simulink model "MdXX_RspOutComm1"  (R2018b)
settings: Solver=FixedStepDiscrete  StartTime=0.0  StopTime=10.0  FixedStep=0.01  RelTol=1e-3
undefined symbols (not defined in the file or in its folder): KeSMSuRspStatHldTm_Val, MdRspLocal2, SrcReqTp1
libraries: simulink x64, RspLib x32
(part 1 of 4)
settings Model: Creator=sn2xws  LastModifiedBy=sn2xws
settings Model: ModifiedHistory=|
  | MD2,MD3不反馈问题修复
  | V2.4.0 Bug 692977 7座 行李箱模式，在调用过程中切换挡位打断调用，返回信号有误
  | 2024.8.19 V3.0.0 Md29反馈逻辑更新
  | //2024.8.20 V3.0.1增加Md53,Md56的反馈
  | 2024.9.13 V3.0.1增加Md2，Md3，Md29被中断的反馈BUG 920831,920834
  | 2024.12.18 V3.8.0 CR 955881 <REQ_MSM_868>
settings DataIOCC: SaveFormat=StructureWithTime
settings OptimizationCC: DefaultParameterBehavior=Inlined  EnhancedBackFolding=on  PassReuseOutputArgsAs=Individual arguments  ZeroExternalMemoryAtStartup=off  ZeroInternalMemoryAtStartup=off  OptimizeBlockOrder=speed  DifferentSizesBufferReuse=on  OptimizationCustomize=off
settings DebuggingCC: ParameterTunabilityLossMsg=error
settings ModelReferenceCC: ModelReferenceNumInstancesAllowed=Single
settings SFSimCC: MATLABDynamicMemAlloc=off
settings RTWCC: SystemTargetFile=autosar.tlc  GenCodeOnly=on  TemplateMakefile=ert_default_tmf  Description=AUTOSAR  GenerateReport=on  IncludeHyperlinkInReport=on  LaunchReport=on  GenerateTraceInfo=on  GenerateTraceReport=on  GenerateTraceReportSl=on  GenerateTraceReportSf=on  GenerateTraceReportEml=on  GenerateCodeMetricsReport=on
settings CodeAppCC: ForceParamTrailComments=on  IgnoreCustomStorageClasses=off  OperatorAnnotations=on  SimulinkDataObjDesc=on  SFDataObjDesc=on  InsertBlockDesc=on
settings STFCustomTargetCC: TargetLangStandard=C99 (ISO)  MultiwordLength=256  ParMdlRefBuildCompliant=on  CompOptLevelCompliant=on  IncludeMdlTerminateFcn=off  CombineOutputUpdateFcns=on  SuppressErrorStatus=on  ERTCustomFileBanners=on  SupportNonFinite=off  SupportComplex=off  SupportContinuousTime=off  SupportNonInlinedSFcns=off  RemoveResetFunc=on  MATLABClassNameForMDSCustomization=Simulink.SoftwareTarget.ERTCustomization  AutosarCompliant=on  UseToolchainInfoCompliant=on  LookupTableObjectStructAxisOrder=2,1,3,4,...  LUTObjectStructOrderEvenSpacing=Size,Table,Breakpoints  SystemTargetFile=autosar.tlc
settings ERTTargetCC: TargetLangStandard=C99 (ISO)  ConcurrentExecutionCompliant=off  IncludeMdlTerminateFcn=off  SuppressErrorStatus=on  SupportNonFinite=off  SupportComplex=off  ModelStepFunctionPrototypeControlCompliant=off  CPPClassGenCompliant=off  AutosarCompliant=on  LookupTableObjectStructAxisOrder=2,1,3,4,...  LUTObjectStructOrderEvenSpacing=Size,Table,Breakpoints  InlinedParameterPlacement=NonHierarchical  ERTCustomFileTemplate=example_file_process.tlc  ERTFilePackagingFormat=Compact

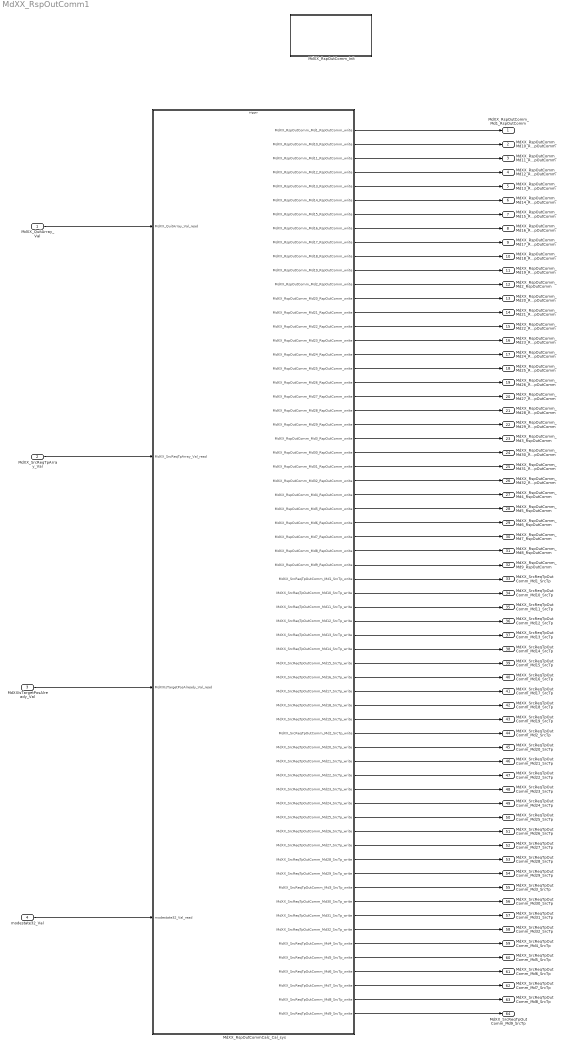
== system MdXX_RspOutComm1 ==
  MdXX_QuitArray_Val : Inport  OutDataTypeStr=Enum: MdRspLocal2  PortDimensions=32
  MdXX_SrcReqTpArray_Val : Inport  Port=2  OutDataTypeStr=Enum: SrcReqTp1  PortDimensions=32
  MdXXIsTargetPosAlready_Val : Inport  Port=3  OutDataTypeStr=uint32  PortDimensions=1
  modestate32_Val : Inport  Port=4  OutDataTypeStr=uint32  PortDimensions=1
  MdXX_RspOutCommCalc_Cal_sys : Subsystem
  MdXX_RspOutComm_Init : Subsystem
  MdXX_RspOutComm_Md1_RspOutComm : Outport  OutDataTypeStr=uint8  PortDimensions=1
  MdXX_RspOutComm_Md10_RspOutComm : Outport  Port=2  OutDataTypeStr=uint8  PortDimensions=1
  MdXX_RspOutComm_Md11_RspOutComm : Outport  Port=3  OutDataTypeStr=uint8  PortDimensions=1
  MdXX_RspOutComm_Md12_RspOutComm : Outport  Port=4  OutDataTypeStr=uint8  PortDimensions=1
  MdXX_RspOutComm_Md13_RspOutComm : Outport  Port=5  OutDataTypeStr=uint8  PortDimensions=1
  MdXX_RspOutComm_Md14_RspOutComm : Outport  Port=6  OutDataTypeStr=uint8  PortDimensions=1
  MdXX_RspOutComm_Md15_RspOutComm : Outport  Port=7  OutDataTypeStr=uint8  PortDimensions=1
  MdXX_RspOutComm_Md16_RspOutComm : Outport  Port=8  OutDataTypeStr=uint8  PortDimensions=1
  MdXX_RspOutComm_Md17_RspOutComm : Outport  Port=9  OutDataTypeStr=uint8  PortDimensions=1
  MdXX_RspOutComm_Md18_RspOutComm : Outport  Port=10  OutDataTypeStr=uint8  PortDimensions=1
  MdXX_RspOutComm_Md19_RspOutComm : Outport  Port=11  OutDataTypeStr=uint8  PortDimensions=1
  MdXX_RspOutComm_Md2_RspOutComm : Outport  Port=12  OutDataTypeStr=uint8  PortDimensions=1
  MdXX_RspOutComm_Md20_RspOutComm : Outport  Port=13  OutDataTypeStr=uint8  PortDimensions=1
  MdXX_RspOutComm_Md21_RspOutComm : Outport  Port=14  OutDataTypeStr=uint8  PortDimensions=1
  MdXX_RspOutComm_Md22_RspOutComm : Outport  Port=15  OutDataTypeStr=uint8  PortDimensions=1
  MdXX_RspOutComm_Md23_RspOutComm : Outport  Port=16  OutDataTypeStr=uint8  PortDimensions=1
  MdXX_RspOutComm_Md24_RspOutComm : Outport  Port=17  OutDataTypeStr=uint8  PortDimensions=1
  MdXX_RspOutComm_Md25_RspOutComm : Outport  Port=18  OutDataTypeStr=uint8  PortDimensions=1
  MdXX_RspOutComm_Md26_RspOutComm : Outport  Port=19  OutDataTypeStr=uint8  PortDimensions=1
  MdXX_RspOutComm_Md27_RspOutComm : Outport  Port=20  OutDataTypeStr=uint8  PortDimensions=1
  MdXX_RspOutComm_Md28_RspOutComm : Outport  Port=21  OutDataTypeStr=uint8  PortDimensions=1
  MdXX_RspOutComm_Md29_RspOutComm : Outport  Port=22  OutDataTypeStr=uint8  PortDimensions=1
  MdXX_RspOutComm_Md3_RspOutComm : Outport  Port=23  OutDataTypeStr=uint8  PortDimensions=1
  MdXX_RspOutComm_Md30_RspOutComm : Outport  Port=24  OutDataTypeStr=uint8  PortDimensions=1
  MdXX_RspOutComm_Md31_RspOutComm : Outport  Port=25  OutDataTypeStr=uint8  PortDimensions=1
  MdXX_RspOutComm_Md32_RspOutComm : Outport  Port=26  OutDataTypeStr=uint8  PortDimensions=1
  MdXX_RspOutComm_Md4_RspOutComm : Outport  Port=27  OutDataTypeStr=uint8  PortDimensions=1
  MdXX_RspOutComm_Md5_RspOutComm : Outport  Port=28  OutDataTypeStr=uint8  PortDimensions=1
  MdXX_RspOutComm_Md6_RspOutComm : Outport  Port=29  OutDataTypeStr=uint8  PortDimensions=1
  MdXX_RspOutComm_Md7_RspOutComm : Outport  Port=30  OutDataTypeStr=uint8  PortDimensions=1
  MdXX_RspOutComm_Md8_RspOutComm : Outport  Port=31  OutDataTypeStr=uint8  PortDimensions=1
  MdXX_RspOutComm_Md9_RspOutComm : Outport  Port=32  OutDataTypeStr=uint8  PortDimensions=1
  MdXX_SrcReqTpOutComm_Md1_SrcTp : Outport  Port=33  OutDataTypeStr=Enum: SrcReqTp1  PortDimensions=1
  MdXX_SrcReqTpOutComm_Md10_SrcTp : Outport  Port=34  OutDataTypeStr=Enum: SrcReqTp1  PortDimensions=1
  MdXX_SrcReqTpOutComm_Md11_SrcTp : Outport  Port=35  OutDataTypeStr=Enum: SrcReqTp1  PortDimensions=1
  MdXX_SrcReqTpOutComm_Md12_SrcTp : Outport  Port=36  OutDataTypeStr=Enum: SrcReqTp1  PortDimensions=1
  MdXX_SrcReqTpOutComm_Md13_SrcTp : Outport  Port=37  OutDataTypeStr=Enum: SrcReqTp1  PortDimensions=1
  MdXX_SrcReqTpOutComm_Md14_SrcTp : Outport  Port=38  OutDataTypeStr=Enum: SrcReqTp1  PortDimensions=1
  MdXX_SrcReqTpOutComm_Md15_SrcTp : Outport  Port=39  OutDataTypeStr=Enum: SrcReqTp1  PortDimensions=1
  MdXX_SrcReqTpOutComm_Md16_SrcTp : Outport  Port=40  OutDataTypeStr=Enum: SrcReqTp1  PortDimensions=1
  MdXX_SrcReqTpOutComm_Md17_SrcTp : Outport  Port=41  OutDataTypeStr=Enum: SrcReqTp1  PortDimensions=1
  MdXX_SrcReqTpOutComm_Md18_SrcTp : Outport  Port=42  OutDataTypeStr=Enum: SrcReqTp1  PortDimensions=1
  MdXX_SrcReqTpOutComm_Md19_SrcTp : Outport  Port=43  OutDataTypeStr=Enum: SrcReqTp1  PortDimensions=1
  MdXX_SrcReqTpOutComm_Md2_SrcTp : Outport  Port=44  OutDataTypeStr=Enum: SrcReqTp1  PortDimensions=1
  MdXX_SrcReqTpOutComm_Md20_SrcTp : Outport  Port=45  OutDataTypeStr=Enum: SrcReqTp1  PortDimensions=1
  MdXX_SrcReqTpOutComm_Md21_SrcTp : Outport  Port=46  OutDataTypeStr=Enum: SrcReqTp1  PortDimensions=1
  MdXX_SrcReqTpOutComm_Md22_SrcTp : Outport  Port=47  OutDataTypeStr=Enum: SrcReqTp1  PortDimensions=1
  MdXX_SrcReqTpOutComm_Md23_SrcTp : Outport  Port=48  OutDataTypeStr=Enum: SrcReqTp1  PortDimensions=1
  MdXX_SrcReqTpOutComm_Md24_SrcTp : Outport  Port=49  OutDataTypeStr=Enum: SrcReqTp1  PortDimensions=1
  MdXX_SrcReqTpOutComm_Md25_SrcTp : Outport  Port=50  OutDataTypeStr=Enum: SrcReqTp1  PortDimensions=1
  MdXX_SrcReqTpOutComm_Md26_SrcTp : Outport  Port=51  OutDataTypeStr=Enum: SrcReqTp1  PortDimensions=1
  MdXX_SrcReqTpOutComm_Md27_SrcTp : Outport  Port=52  OutDataTypeStr=Enum: SrcReqTp1  PortDimensions=1
  MdXX_SrcReqTpOutComm_Md28_SrcTp : Outport  Port=53  OutDataTypeStr=Enum: SrcReqTp1  PortDimensions=1
  MdXX_SrcReqTpOutComm_Md29_SrcTp : Outport  Port=54  OutDataTypeStr=Enum: SrcReqTp1  PortDimensions=1
  MdXX_SrcReqTpOutComm_Md3_SrcTp : Outport  Port=55  OutDataTypeStr=Enum: SrcReqTp1  PortDimensions=1
  MdXX_SrcReqTpOutComm_Md30_SrcTp : Outport  Port=56  OutDataTypeStr=Enum: SrcReqTp1  PortDimensions=1
  MdXX_SrcReqTpOutComm_Md31_SrcTp : Outport  Port=57  OutDataTypeStr=Enum: SrcReqTp1  PortDimensions=1
  MdXX_SrcReqTpOutComm_Md32_SrcTp : Outport  Port=58  OutDataTypeStr=Enum: SrcReqTp1  PortDimensions=1
  MdXX_SrcReqTpOutComm_Md4_SrcTp : Outport  Port=59  OutDataTypeStr=Enum: SrcReqTp1  PortDimensions=1
  MdXX_SrcReqTpOutComm_Md5_SrcTp : Outport  Port=60  OutDataTypeStr=Enum: SrcReqTp1  PortDimensions=1
  MdXX_SrcReqTpOutComm_Md6_SrcTp : Outport  Port=61  OutDataTypeStr=Enum: SrcReqTp1  PortDimensions=1
  MdXX_SrcReqTpOutComm_Md7_SrcTp : Outport  Port=62  OutDataTypeStr=Enum: SrcReqTp1  PortDimensions=1
  MdXX_SrcReqTpOutComm_Md8_SrcTp : Outport  Port=63  OutDataTypeStr=Enum: SrcReqTp1  PortDimensions=1
  MdXX_SrcReqTpOutComm_Md9_SrcTp : Outport  Port=64  OutDataTypeStr=Enum: SrcReqTp1  PortDimensions=1
  wires:
  MdXX_QuitArray_Val/1 -> MdXX_RspOutCommCalc_Cal_sys/1(MdXX_QuitArray_Val_read)
  MdXX_SrcReqTpArray_Val/1 -> MdXX_RspOutCommCalc_Cal_sys/2(MdXX_SrcReqTpArray_Val_read)
  modestate32_Val/1 -> MdXX_RspOutCommCalc_Cal_sys/4(modestate32_Val_read)
  MdXXIsTargetPosAlready_Val/1 -> MdXX_RspOutCommCalc_Cal_sys/3(MdXXIsTargetPosAlready_Val_read)
  MdXX_RspOutCommCalc_Cal_sys/1(MdXX_RspOutComm_Md1_RspOutComm_write) -> MdXX_RspOutComm_Md1_RspOutComm/1
  MdXX_RspOutCommCalc_Cal_sys/2(MdXX_RspOutComm_Md10_RspOutComm_write) -> MdXX_RspOutComm_Md10_RspOutComm/1
  MdXX_RspOutCommCalc_Cal_sys/3(MdXX_RspOutComm_Md11_RspOutComm_write) -> MdXX_RspOutComm_Md11_RspOutComm/1
  MdXX_RspOutCommCalc_Cal_sys/4(MdXX_RspOutComm_Md12_RspOutComm_write) -> MdXX_RspOutComm_Md12_RspOutComm/1
  MdXX_RspOutCommCalc_Cal_sys/5(MdXX_RspOutComm_Md13_RspOutComm_write) -> MdXX_RspOutComm_Md13_RspOutComm/1
  MdXX_RspOutCommCalc_Cal_sys/6(MdXX_RspOutComm_Md14_RspOutComm_write) -> MdXX_RspOutComm_Md14_RspOutComm/1
  MdXX_RspOutCommCalc_Cal_sys/7(MdXX_RspOutComm_Md15_RspOutComm_write) -> MdXX_RspOutComm_Md15_RspOutComm/1
  MdXX_RspOutCommCalc_Cal_sys/8(MdXX_RspOutComm_Md16_RspOutComm_write) -> MdXX_RspOutComm_Md16_RspOutComm/1
  MdXX_RspOutCommCalc_Cal_sys/9(MdXX_RspOutComm_Md17_RspOutComm_write) -> MdXX_RspOutComm_Md17_RspOutComm/1
  MdXX_RspOutCommCalc_Cal_sys/10(MdXX_RspOutComm_Md18_RspOutComm_write) -> MdXX_RspOutComm_Md18_RspOutComm/1
  MdXX_RspOutCommCalc_Cal_sys/11(MdXX_RspOutComm_Md19_RspOutComm_write) -> MdXX_RspOutComm_Md19_RspOutComm/1
  MdXX_RspOutCommCalc_Cal_sys/12(MdXX_RspOutComm_Md2_RspOutComm_write) -> MdXX_RspOutComm_Md2_RspOutComm/1
  MdXX_RspOutCommCalc_Cal_sys/13(MdXX_RspOutComm_Md20_RspOutComm_write) -> MdXX_RspOutComm_Md20_RspOutComm/1
  MdXX_RspOutCommCalc_Cal_sys/14(MdXX_RspOutComm_Md21_RspOutComm_write) -> MdXX_RspOutComm_Md21_RspOutComm/1
  MdXX_RspOutCommCalc_Cal_sys/15(MdXX_RspOutComm_Md22_RspOutComm_write) -> MdXX_RspOutComm_Md22_RspOutComm/1
  MdXX_RspOutCommCalc_Cal_sys/16(MdXX_RspOutComm_Md23_RspOutComm_write) -> MdXX_RspOutComm_Md23_RspOutComm/1
  MdXX_RspOutCommCalc_Cal_sys/17(MdXX_RspOutComm_Md24_RspOutComm_write) -> MdXX_RspOutComm_Md24_RspOutComm/1
  MdXX_RspOutCommCalc_Cal_sys/18(MdXX_RspOutComm_Md25_RspOutComm_write) -> MdXX_RspOutComm_Md25_RspOutComm/1
  MdXX_RspOutCommCalc_Cal_sys/19(MdXX_RspOutComm_Md26_RspOutComm_write) -> MdXX_RspOutComm_Md26_RspOutComm/1
  MdXX_RspOutCommCalc_Cal_sys/20(MdXX_RspOutComm_Md27_RspOutComm_write) -> MdXX_RspOutComm_Md27_RspOutComm/1
  MdXX_RspOutCommCalc_Cal_sys/21(MdXX_RspOutComm_Md28_RspOutComm_write) -> MdXX_RspOutComm_Md28_RspOutComm/1
  MdXX_RspOutCommCalc_Cal_sys/22(MdXX_RspOutComm_Md29_RspOutComm_write) -> MdXX_RspOutComm_Md29_RspOutComm/1
  MdXX_RspOutCommCalc_Cal_sys/23(MdXX_RspOutComm_Md3_RspOutComm_write) -> MdXX_RspOutComm_Md3_RspOutComm/1
  MdXX_RspOutCommCalc_Cal_sys/24(MdXX_RspOutComm_Md30_RspOutComm_write) -> MdXX_RspOutComm_Md30_RspOutComm/1
  MdXX_RspOutCommCalc_Cal_sys/25(MdXX_RspOutComm_Md31_RspOutComm_write) -> MdXX_RspOutComm_Md31_RspOutComm/1
  MdXX_RspOutCommCalc_Cal_sys/26(MdXX_RspOutComm_Md32_RspOutComm_write) -> MdXX_RspOutComm_Md32_RspOutComm/1
  MdXX_RspOutCommCalc_Cal_sys/27(MdXX_RspOutComm_Md4_RspOutComm_write) -> MdXX_RspOutComm_Md4_RspOutComm/1
  MdXX_RspOutCommCalc_Cal_sys/28(MdXX_RspOutComm_Md5_RspOutComm_write) -> MdXX_RspOutComm_Md5_RspOutComm/1
  MdXX_RspOutCommCalc_Cal_sys/29(MdXX_RspOutComm_Md6_RspOutComm_write) -> MdXX_RspOutComm_Md6_RspOutComm/1
  MdXX_RspOutCommCalc_Cal_sys/30(MdXX_RspOutComm_Md7_RspOutComm_write) -> MdXX_RspOutComm_Md7_RspOutComm/1
  MdXX_RspOutCommCalc_Cal_sys/31(MdXX_RspOutComm_Md8_RspOutComm_write) -> MdXX_RspOutComm_Md8_RspOutComm/1
  MdXX_RspOutCommCalc_Cal_sys/32(MdXX_RspOutComm_Md9_RspOutComm_write) -> MdXX_RspOutComm_Md9_RspOutComm/1
  MdXX_RspOutCommCalc_Cal_sys/33(MdXX_SrcReqTpOutComm_Md1_SrcTp_write) -> MdXX_SrcReqTpOutComm_Md1_SrcTp/1
  MdXX_RspOutCommCalc_Cal_sys/34(MdXX_SrcReqTpOutComm_Md10_SrcTp_write) -> MdXX_SrcReqTpOutComm_Md10_SrcTp/1
  MdXX_RspOutCommCalc_Cal_sys/35(MdXX_SrcReqTpOutComm_Md11_SrcTp_write) -> MdXX_SrcReqTpOutComm_Md11_SrcTp/1
  MdXX_RspOutCommCalc_Cal_sys/36(MdXX_SrcReqTpOutComm_Md12_SrcTp_write) -> MdXX_SrcReqTpOutComm_Md12_SrcTp/1
  MdXX_RspOutCommCalc_Cal_sys/37(MdXX_SrcReqTpOutComm_Md13_SrcTp_write) -> MdXX_SrcReqTpOutComm_Md13_SrcTp/1
  MdXX_RspOutCommCalc_Cal_sys/38(MdXX_SrcReqTpOutComm_Md14_SrcTp_write) -> MdXX_SrcReqTpOutComm_Md14_SrcTp/1
  MdXX_RspOutCommCalc_Cal_sys/39(MdXX_SrcReqTpOutComm_Md15_SrcTp_write) -> MdXX_SrcReqTpOutComm_Md15_SrcTp/1
  MdXX_RspOutCommCalc_Cal_sys/40(MdXX_SrcReqTpOutComm_Md16_SrcTp_write) -> MdXX_SrcReqTpOutComm_Md16_SrcTp/1
  MdXX_RspOutCommCalc_Cal_sys/41(MdXX_SrcReqTpOutComm_Md17_SrcTp_write) -> MdXX_SrcReqTpOutComm_Md17_SrcTp/1
  MdXX_RspOutCommCalc_Cal_sys/42(MdXX_SrcReqTpOutComm_Md18_SrcTp_write) -> MdXX_SrcReqTpOutComm_Md18_SrcTp/1
  MdXX_RspOutCommCalc_Cal_sys/43(MdXX_SrcReqTpOutComm_Md19_SrcTp_write) -> MdXX_SrcReqTpOutComm_Md19_SrcTp/1
  MdXX_RspOutCommCalc_Cal_sys/44(MdXX_SrcReqTpOutComm_Md2_SrcTp_write) -> MdXX_SrcReqTpOutComm_Md2_SrcTp/1
  MdXX_RspOutCommCalc_Cal_sys/45(MdXX_SrcReqTpOutComm_Md20_SrcTp_write) -> MdXX_SrcReqTpOutComm_Md20_SrcTp/1
  MdXX_RspOutCommCalc_Cal_sys/46(MdXX_SrcReqTpOutComm_Md21_SrcTp_write) -> MdXX_SrcReqTpOutComm_Md21_SrcTp/1
  MdXX_RspOutCommCalc_Cal_sys/47(MdXX_SrcReqTpOutComm_Md22_SrcTp_write) -> MdXX_SrcReqTpOutComm_Md22_SrcTp/1
  MdXX_RspOutCommCalc_Cal_sys/48(MdXX_SrcReqTpOutComm_Md23_SrcTp_write) -> MdXX_SrcReqTpOutComm_Md23_SrcTp/1
  MdXX_RspOutCommCalc_Cal_sys/49(MdXX_SrcReqTpOutComm_Md24_SrcTp_write) -> MdXX_SrcReqTpOutComm_Md24_SrcTp/1
  MdXX_RspOutCommCalc_Cal_sys/50(MdXX_SrcReqTpOutComm_Md25_SrcTp_write) -> MdXX_SrcReqTpOutComm_Md25_SrcTp/1
  MdXX_RspOutCommCalc_Cal_sys/51(MdXX_SrcReqTpOutComm_Md26_SrcTp_write) -> MdXX_SrcReqTpOutComm_Md26_SrcTp/1
  MdXX_RspOutCommCalc_Cal_sys/52(MdXX_SrcReqTpOutComm_Md27_SrcTp_write) -> MdXX_SrcReqTpOutComm_Md27_SrcTp/1
  MdXX_RspOutCommCalc_Cal_sys/53(MdXX_SrcReqTpOutComm_Md28_SrcTp_write) -> MdXX_SrcReqTpOutComm_Md28_SrcTp/1
  MdXX_RspOutCommCalc_Cal_sys/54(MdXX_SrcReqTpOutComm_Md29_SrcTp_write) -> MdXX_SrcReqTpOutComm_Md29_SrcTp/1
  MdXX_RspOutCommCalc_Cal_sys/55(MdXX_SrcReqTpOutComm_Md3_SrcTp_write) -> MdXX_SrcReqTpOutComm_Md3_SrcTp/1
  MdXX_RspOutCommCalc_Cal_sys/56(MdXX_SrcReqTpOutComm_Md30_SrcTp_write) -> MdXX_SrcReqTpOutComm_Md30_SrcTp/1
  MdXX_RspOutCommCalc_Cal_sys/57(MdXX_SrcReqTpOutComm_Md31_SrcTp_write) -> MdXX_SrcReqTpOutComm_Md31_SrcTp/1
  MdXX_RspOutCommCalc_Cal_sys/58(MdXX_SrcReqTpOutComm_Md32_SrcTp_write) -> MdXX_SrcReqTpOutComm_Md32_SrcTp/1
  MdXX_RspOutCommCalc_Cal_sys/59(MdXX_SrcReqTpOutComm_Md4_SrcTp_write) -> MdXX_SrcReqTpOutComm_Md4_SrcTp/1
  MdXX_RspOutCommCalc_Cal_sys/60(MdXX_SrcReqTpOutComm_Md5_SrcTp_write) -> MdXX_SrcReqTpOutComm_Md5_SrcTp/1
  MdXX_RspOutCommCalc_Cal_sys/61(MdXX_SrcReqTpOutComm_Md6_SrcTp_write) -> MdXX_SrcReqTpOutComm_Md6_SrcTp/1
  MdXX_RspOutCommCalc_Cal_sys/62(MdXX_SrcReqTpOutComm_Md7_SrcTp_write) -> MdXX_SrcReqTpOutComm_Md7_SrcTp/1
  MdXX_RspOutCommCalc_Cal_sys/63(MdXX_SrcReqTpOutComm_Md8_SrcTp_write) -> MdXX_SrcReqTpOutComm_Md8_SrcTp/1
  MdXX_RspOutCommCalc_Cal_sys/64(MdXX_SrcReqTpOutComm_Md9_SrcTp_write) -> MdXX_SrcReqTpOutComm_Md9_SrcTp/1

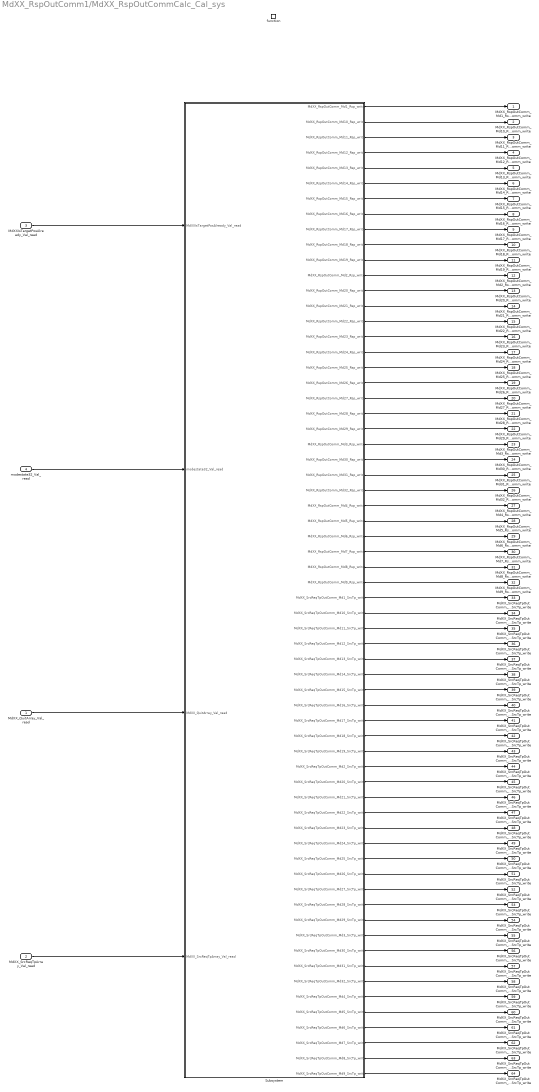
== system MdXX_RspOutComm1/MdXX_RspOutCommCalc_Cal_sys ==
  MdXX_QuitArray_Val_read : Inport
  MdXX_SrcReqTpArray_Val_read : Inport  Port=2
  MdXXIsTargetPosAlready_Val_read : Inport  Port=3
  modestate32_Val_read : Inport  Port=4
  function : TriggerPort  TriggerType=function-call  IsSimulinkFunction=on  FunctionName=MdXX_RspOutCommCalc_Cal  VariantControl=(inherit)
  Subsystem : Subsystem
  MdXX_RspOutComm_Md1_RspOutComm_write : Outport  InitialOutput=0
  MdXX_RspOutComm_Md10_RspOutComm_write : Outport  Port=2  InitialOutput=0
  MdXX_RspOutComm_Md11_RspOutComm_write : Outport  Port=3  InitialOutput=0
  MdXX_RspOutComm_Md12_RspOutComm_write : Outport  Port=4  InitialOutput=0
  MdXX_RspOutComm_Md13_RspOutComm_write : Outport  Port=5  InitialOutput=0
  MdXX_RspOutComm_Md14_RspOutComm_write : Outport  Port=6  InitialOutput=0
  MdXX_RspOutComm_Md15_RspOutComm_write : Outport  Port=7  InitialOutput=0
  MdXX_RspOutComm_Md16_RspOutComm_write : Outport  Port=8  InitialOutput=0
  MdXX_RspOutComm_Md17_RspOutComm_write : Outport  Port=9  InitialOutput=0
  MdXX_RspOutComm_Md18_RspOutComm_write : Outport  Port=10  InitialOutput=0
  MdXX_RspOutComm_Md19_RspOutComm_write : Outport  Port=11  InitialOutput=0
  MdXX_RspOutComm_Md2_RspOutComm_write : Outport  Port=12  InitialOutput=0
  MdXX_RspOutComm_Md20_RspOutComm_write : Outport  Port=13  InitialOutput=0
  MdXX_RspOutComm_Md21_RspOutComm_write : Outport  Port=14  InitialOutput=0
  MdXX_RspOutComm_Md22_RspOutComm_write : Outport  Port=15  InitialOutput=0
  MdXX_RspOutComm_Md23_RspOutComm_write : Outport  Port=16  InitialOutput=0
  MdXX_RspOutComm_Md24_RspOutComm_write : Outport  Port=17  InitialOutput=0
  MdXX_RspOutComm_Md25_RspOutComm_write : Outport  Port=18  InitialOutput=0
  MdXX_RspOutComm_Md26_RspOutComm_write : Outport  Port=19  InitialOutput=0
  MdXX_RspOutComm_Md27_RspOutComm_write : Outport  Port=20  InitialOutput=0
  MdXX_RspOutComm_Md28_RspOutComm_write : Outport  Port=21  InitialOutput=0
  MdXX_RspOutComm_Md29_RspOutComm_write : Outport  Port=22  InitialOutput=0
  MdXX_RspOutComm_Md3_RspOutComm_write : Outport  Port=23  InitialOutput=0
  MdXX_RspOutComm_Md30_RspOutComm_write : Outport  Port=24  InitialOutput=0
  MdXX_RspOutComm_Md31_RspOutComm_write : Outport  Port=25  InitialOutput=0
  MdXX_RspOutComm_Md32_RspOutComm_write : Outport  Port=26  InitialOutput=0
  MdXX_RspOutComm_Md4_RspOutComm_write : Outport  Port=27  InitialOutput=0
  MdXX_RspOutComm_Md5_RspOutComm_write : Outport  Port=28  InitialOutput=0
  MdXX_RspOutComm_Md6_RspOutComm_write : Outport  Port=29  InitialOutput=0
  MdXX_RspOutComm_Md7_RspOutComm_write : Outport  Port=30  InitialOutput=0
  MdXX_RspOutComm_Md8_RspOutComm_write : Outport  Port=31  InitialOutput=0
  MdXX_RspOutComm_Md9_RspOutComm_write : Outport  Port=32  InitialOutput=0
  MdXX_SrcReqTpOutComm_Md1_SrcTp_write : Outport  Port=33  InitialOutput=SrcReqTp1.SrcReqTp_None
  MdXX_SrcReqTpOutComm_Md10_SrcTp_write : Outport  Port=34  InitialOutput=SrcReqTp1.SrcReqTp_None
  MdXX_SrcReqTpOutComm_Md11_SrcTp_write : Outport  Port=35  InitialOutput=SrcReqTp1.SrcReqTp_None
  MdXX_SrcReqTpOutComm_Md12_SrcTp_write : Outport  Port=36  InitialOutput=SrcReqTp1.SrcReqTp_None
  MdXX_SrcReqTpOutComm_Md13_SrcTp_write : Outport  Port=37  InitialOutput=SrcReqTp1.SrcReqTp_None
  MdXX_SrcReqTpOutComm_Md14_SrcTp_write : Outport  Port=38  InitialOutput=SrcReqTp1.SrcReqTp_None
  MdXX_SrcReqTpOutComm_Md15_SrcTp_write : Outport  Port=39  InitialOutput=SrcReqTp1.SrcReqTp_None
  MdXX_SrcReqTpOutComm_Md16_SrcTp_write : Outport  Port=40  InitialOutput=SrcReqTp1.SrcReqTp_None
  MdXX_SrcReqTpOutComm_Md17_SrcTp_write : Outport  Port=41  InitialOutput=SrcReqTp1.SrcReqTp_None
  MdXX_SrcReqTpOutComm_Md18_SrcTp_write : Outport  Port=42  InitialOutput=SrcReqTp1.SrcReqTp_None
  MdXX_SrcReqTpOutComm_Md19_SrcTp_write : Outport  Port=43  InitialOutput=SrcReqTp1.SrcReqTp_None
  MdXX_SrcReqTpOutComm_Md2_SrcTp_write : Outport  Port=44  InitialOutput=SrcReqTp1.SrcReqTp_None
  MdXX_SrcReqTpOutComm_Md20_SrcTp_write : Outport  Port=45  InitialOutput=SrcReqTp1.SrcReqTp_None
  MdXX_SrcReqTpOutComm_Md21_SrcTp_write : Outport  Port=46  InitialOutput=SrcReqTp1.SrcReqTp_None
  MdXX_SrcReqTpOutComm_Md22_SrcTp_write : Outport  Port=47  InitialOutput=SrcReqTp1.SrcReqTp_None
  MdXX_SrcReqTpOutComm_Md23_SrcTp_write : Outport  Port=48  InitialOutput=SrcReqTp1.SrcReqTp_None
  MdXX_SrcReqTpOutComm_Md24_SrcTp_write : Outport  Port=49  InitialOutput=SrcReqTp1.SrcReqTp_None
  MdXX_SrcReqTpOutComm_Md25_SrcTp_write : Outport  Port=50  InitialOutput=SrcReqTp1.SrcReqTp_None
  MdXX_SrcReqTpOutComm_Md26_SrcTp_write : Outport  Port=51  InitialOutput=SrcReqTp1.SrcReqTp_None
  MdXX_SrcReqTpOutComm_Md27_SrcTp_write : Outport  Port=52  InitialOutput=SrcReqTp1.SrcReqTp_None
  MdXX_SrcReqTpOutComm_Md28_SrcTp_write : Outport  Port=53  InitialOutput=SrcReqTp1.SrcReqTp_None
  MdXX_SrcReqTpOutComm_Md29_SrcTp_write : Outport  Port=54  InitialOutput=SrcReqTp1.SrcReqTp_None
  MdXX_SrcReqTpOutComm_Md3_SrcTp_write : Outport  Port=55  InitialOutput=SrcReqTp1.SrcReqTp_None
  MdXX_SrcReqTpOutComm_Md30_SrcTp_write : Outport  Port=56  InitialOutput=SrcReqTp1.SrcReqTp_None
  MdXX_SrcReqTpOutComm_Md31_SrcTp_write : Outport  Port=57  InitialOutput=SrcReqTp1.SrcReqTp_None
  MdXX_SrcReqTpOutComm_Md32_SrcTp_write : Outport  Port=58  InitialOutput=SrcReqTp1.SrcReqTp_None
  MdXX_SrcReqTpOutComm_Md4_SrcTp_write : Outport  Port=59  InitialOutput=SrcReqTp1.SrcReqTp_None
  MdXX_SrcReqTpOutComm_Md5_SrcTp_write : Outport  Port=60  InitialOutput=SrcReqTp1.SrcReqTp_None
  MdXX_SrcReqTpOutComm_Md6_SrcTp_write : Outport  Port=61  InitialOutput=SrcReqTp1.SrcReqTp_None
  MdXX_SrcReqTpOutComm_Md7_SrcTp_write : Outport  Port=62  InitialOutput=SrcReqTp1.SrcReqTp_None
  MdXX_SrcReqTpOutComm_Md8_SrcTp_write : Outport  Port=63  InitialOutput=SrcReqTp1.SrcReqTp_None
  MdXX_SrcReqTpOutComm_Md9_SrcTp_write : Outport  Port=64  InitialOutput=SrcReqTp1.SrcReqTp_None
  wires:
  MdXXIsTargetPosAlready_Val_read/1 -> Subsystem/1(MdXXIsTargetPosAlready_Val_read)
  modestate32_Val_read/1 -> Subsystem/2(modestate32_Val_read)
  MdXX_QuitArray_Val_read/1 -> Subsystem/3(MdXX_QuitArray_Val_read)
  MdXX_SrcReqTpArray_Val_read/1 -> Subsystem/4(MdXX_SrcReqTpArray_Val_read)
  Subsystem/17(MdXX_RspOutComm_Md24_Rsp_write) -> MdXX_RspOutComm_Md24_RspOutComm_write/1
  Subsystem/15(MdXX_RspOutComm_Md22_Rsp_write) -> MdXX_RspOutComm_Md22_RspOutComm_write/1
  Subsystem/16(MdXX_RspOutComm_Md23_Rsp_write) -> MdXX_RspOutComm_Md23_RspOutComm_write/1
  Subsystem/18(MdXX_RspOutComm_Md25_Rsp_write) -> MdXX_RspOutComm_Md25_RspOutComm_write/1
  Subsystem/19(MdXX_RspOutComm_Md26_Rsp_write) -> MdXX_RspOutComm_Md26_RspOutComm_write/1
  Subsystem/13(MdXX_RspOutComm_Md20_Rsp_write) -> MdXX_RspOutComm_Md20_RspOutComm_write/1
  Subsystem/14(MdXX_RspOutComm_Md21_Rsp_write) -> MdXX_RspOutComm_Md21_RspOutComm_write/1
  Subsystem/20(MdXX_RspOutComm_Md27_Rsp_write) -> MdXX_RspOutComm_Md27_RspOutComm_write/1
  Subsystem/21(MdXX_RspOutComm_Md28_Rsp_write) -> MdXX_RspOutComm_Md28_RspOutComm_write/1
  Subsystem/12(MdXX_RspOutComm_Md2_Rsp_write) -> MdXX_RspOutComm_Md2_RspOutComm_write/1
  Subsystem/22(MdXX_RspOutComm_Md29_Rsp_write) -> MdXX_RspOutComm_Md29_RspOutComm_write/1
  Subsystem/10(MdXX_RspOutComm_Md18_Rsp_write) -> MdXX_RspOutComm_Md18_RspOutComm_write/1
  Subsystem/11(MdXX_RspOutComm_Md19_Rsp_write) -> MdXX_RspOutComm_Md19_RspOutComm_write/1
  Subsystem/23(MdXX_RspOutComm_Md3_Rsp_write) -> MdXX_RspOutComm_Md3_RspOutComm_write/1
  Subsystem/24(MdXX_RspOutComm_Md30_Rsp_write) -> MdXX_RspOutComm_Md30_RspOutComm_write/1
  Subsystem/8(MdXX_RspOutComm_Md16_Rsp_write) -> MdXX_RspOutComm_Md16_RspOutComm_write/1
  Subsystem/9(MdXX_RspOutComm_Md17_Rsp_write) -> MdXX_RspOutComm_Md17_RspOutComm_write/1
  Subsystem/25(MdXX_RspOutComm_Md31_Rsp_write) -> MdXX_RspOutComm_Md31_RspOutComm_write/1
  Subsystem/26(MdXX_RspOutComm_Md32_Rsp_write) -> MdXX_RspOutComm_Md32_RspOutComm_write/1
  Subsystem/7(MdXX_RspOutComm_Md15_Rsp_write) -> MdXX_RspOutComm_Md15_RspOutComm_write/1
  Subsystem/27(MdXX_RspOutComm_Md4_Rsp_write) -> MdXX_RspOutComm_Md4_RspOutComm_write/1
  Subsystem/5(MdXX_RspOutComm_Md13_Rsp_write) -> MdXX_RspOutComm_Md13_RspOutComm_write/1
  Subsystem/6(MdXX_RspOutComm_Md14_Rsp_write) -> MdXX_RspOutComm_Md14_RspOutComm_write/1
  Subsystem/28(MdXX_RspOutComm_Md5_Rsp_write) -> MdXX_RspOutComm_Md5_RspOutComm_write/1
  Subsystem/29(MdXX_RspOutComm_Md6_Rsp_write) -> MdXX_RspOutComm_Md6_RspOutComm_write/1
  Subsystem/3(MdXX_RspOutComm_Md11_Rsp_write) -> MdXX_RspOutComm_Md11_RspOutComm_write/1
  Subsystem/4(MdXX_RspOutComm_Md12_Rsp_write) -> MdXX_RspOutComm_Md12_RspOutComm_write/1
  Subsystem/30(MdXX_RspOutComm_Md7_Rsp_write) -> MdXX_RspOutComm_Md7_RspOutComm_write/1
  Subsystem/31(MdXX_RspOutComm_Md8_Rsp_write) -> MdXX_RspOutComm_Md8_RspOutComm_write/1
  Subsystem/2(MdXX_RspOutComm_Md10_Rsp_write) -> MdXX_RspOutComm_Md10_RspOutComm_write/1
  Subsystem/32(MdXX_RspOutComm_Md9_Rsp_write) -> MdXX_RspOutComm_Md9_RspOutComm_write/1
  Subsystem/1(MdXX_RspOutComm_Md1_Rsp_write) -> MdXX_RspOutComm_Md1_RspOutComm_write/1
  Subsystem/33(MdXX_SrcReqTpOutComm_Md1_SrcTp_write) -> MdXX_SrcReqTpOutComm_Md1_SrcTp_write/1
  Subsystem/34(MdXX_SrcReqTpOutComm_Md10_SrcTp_write) -> MdXX_SrcReqTpOutComm_Md10_SrcTp_write/1
  Subsystem/35(MdXX_SrcReqTpOutComm_Md11_SrcTp_write) -> MdXX_SrcReqTpOutComm_Md11_SrcTp_write/1
  Subsystem/36(MdXX_SrcReqTpOutComm_Md12_SrcTp_write) -> MdXX_SrcReqTpOutComm_Md12_SrcTp_write/1
  Subsystem/37(MdXX_SrcReqTpOutComm_Md13_SrcTp_write) -> MdXX_SrcReqTpOutComm_Md13_SrcTp_write/1
  Subsystem/38(MdXX_SrcReqTpOutComm_Md14_SrcTp_write) -> MdXX_SrcReqTpOutComm_Md14_SrcTp_write/1
  Subsystem/39(MdXX_SrcReqTpOutComm_Md15_SrcTp_write) -> MdXX_SrcReqTpOutComm_Md15_SrcTp_write/1
  Subsystem/40(MdXX_SrcReqTpOutComm_Md16_SrcTp_write) -> MdXX_SrcReqTpOutComm_Md16_SrcTp_write/1
  Subsystem/41(MdXX_SrcReqTpOutComm_Md17_SrcTp_write) -> MdXX_SrcReqTpOutComm_Md17_SrcTp_write/1
  Subsystem/42(MdXX_SrcReqTpOutComm_Md18_SrcTp_write) -> MdXX_SrcReqTpOutComm_Md18_SrcTp_write/1
  Subsystem/43(MdXX_SrcReqTpOutComm_Md19_SrcTp_write) -> MdXX_SrcReqTpOutComm_Md19_SrcTp_write/1
  Subsystem/44(MdXX_SrcReqTpOutComm_Md2_SrcTp_write) -> MdXX_SrcReqTpOutComm_Md2_SrcTp_write/1
  Subsystem/45(MdXX_SrcReqTpOutComm_Md20_SrcTp_write) -> MdXX_SrcReqTpOutComm_Md20_SrcTp_write/1
  Subsystem/46(MdXX_SrcReqTpOutComm_Md21_SrcTp_write) -> MdXX_SrcReqTpOutComm_Md21_SrcTp_write/1
  Subsystem/47(MdXX_SrcReqTpOutComm_Md22_SrcTp_write) -> MdXX_SrcReqTpOutComm_Md22_SrcTp_write/1
  Subsystem/48(MdXX_SrcReqTpOutComm_Md23_SrcTp_write) -> MdXX_SrcReqTpOutComm_Md23_SrcTp_write/1
  Subsystem/49(MdXX_SrcReqTpOutComm_Md24_SrcTp_write) -> MdXX_SrcReqTpOutComm_Md24_SrcTp_write/1
  Subsystem/50(MdXX_SrcReqTpOutComm_Md25_SrcTp_write) -> MdXX_SrcReqTpOutComm_Md25_SrcTp_write/1
  Subsystem/51(MdXX_SrcReqTpOutComm_Md26_SrcTp_write) -> MdXX_SrcReqTpOutComm_Md26_SrcTp_write/1
  Subsystem/52(MdXX_SrcReqTpOutComm_Md27_SrcTp_write) -> MdXX_SrcReqTpOutComm_Md27_SrcTp_write/1
  Subsystem/53(MdXX_SrcReqTpOutComm_Md28_SrcTp_write) -> MdXX_SrcReqTpOutComm_Md28_SrcTp_write/1
  Subsystem/54(MdXX_SrcReqTpOutComm_Md29_SrcTp_write) -> MdXX_SrcReqTpOutComm_Md29_SrcTp_write/1
  Subsystem/55(MdXX_SrcReqTpOutComm_Md3_SrcTp_write) -> MdXX_SrcReqTpOutComm_Md3_SrcTp_write/1
  Subsystem/56(MdXX_SrcReqTpOutComm_Md30_SrcTp_write) -> MdXX_SrcReqTpOutComm_Md30_SrcTp_write/1
  Subsystem/57(MdXX_SrcReqTpOutComm_Md31_SrcTp_write) -> MdXX_SrcReqTpOutComm_Md31_SrcTp_write/1
  Subsystem/58(MdXX_SrcReqTpOutComm_Md32_SrcTp_write) -> MdXX_SrcReqTpOutComm_Md32_SrcTp_write/1
  Subsystem/59(MdXX_SrcReqTpOutComm_Md4_SrcTp_write) -> MdXX_SrcReqTpOutComm_Md4_SrcTp_write/1
  Subsystem/60(MdXX_SrcReqTpOutComm_Md5_SrcTp_write) -> MdXX_SrcReqTpOutComm_Md5_SrcTp_write/1
  Subsystem/61(MdXX_SrcReqTpOutComm_Md6_SrcTp_write) -> MdXX_SrcReqTpOutComm_Md6_SrcTp_write/1
  Subsystem/62(MdXX_SrcReqTpOutComm_Md7_SrcTp_write) -> MdXX_SrcReqTpOutComm_Md7_SrcTp_write/1
  Subsystem/63(MdXX_SrcReqTpOutComm_Md8_SrcTp_write) -> MdXX_SrcReqTpOutComm_Md8_SrcTp_write/1
  Subsystem/64(MdXX_SrcReqTpOutComm_Md9_SrcTp_write) -> MdXX_SrcReqTpOutComm_Md9_SrcTp_write/1

== system MdXX_RspOutComm1/MdXX_RspOutComm_Init ==
  Event Listener : EventListener  EventName=reset
